simulink model "Rozmyty_fuzzy_controler"  (R2017b)
settings: Solver=ode1  StartTime=0.0  StopTime=4  FixedStep=0.001  RelTol=1e-3
values from neighbouring files (symbols this model uses):
  Te = 0.001    [Dane_rozmyte.m]
  Tm = 0.2    [Dane_rozmyte.m]
libraries: fuzblock x6
settings Model: Creator=kamil  LastModifiedBy=kamil

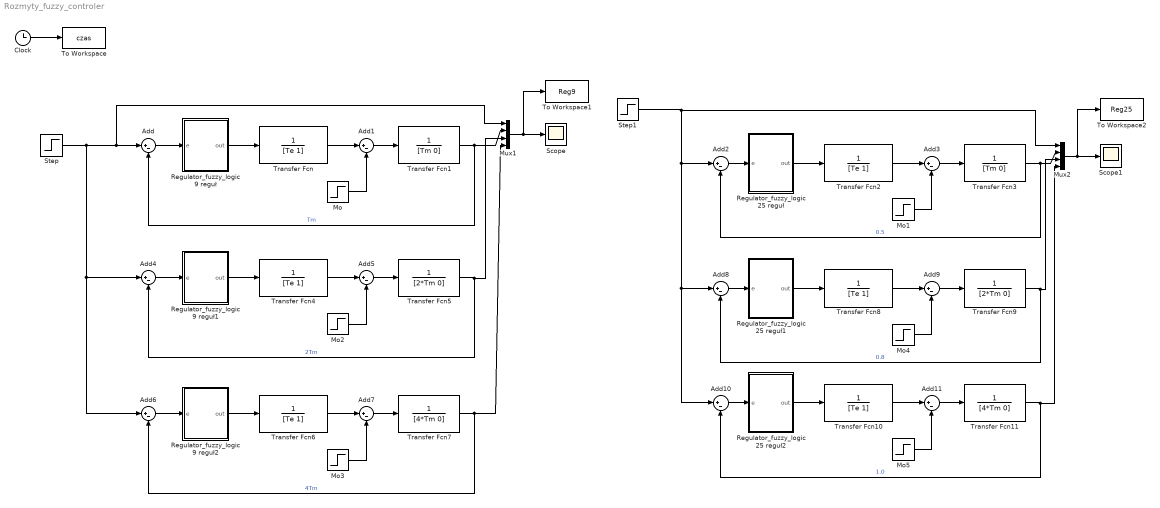
== system Rozmyty_fuzzy_controler ==
  Add{,1..11} (12 alike) : Sum  Inputs=|+-
  Clock : Clock
  Mo{,1..5} (6 alike) : Step  Time=2  After=0.5  SampleTime=0
  Mux1 : Mux
  Mux2 : Mux
  Regulator_fuzzy_logic 25 reguł : Subsystem
  Regulator_fuzzy_logic 25 reguł1 : Subsystem
  Regulator_fuzzy_logic 25 reguł2 : Subsystem
  Regulator_fuzzy_logic 9 reguł : Subsystem
  Regulator_fuzzy_logic 9 reguł1 : Subsystem
  Regulator_fuzzy_logic 9 reguł2 : Subsystem
  Scope : Scope
  Scope1 : Scope
  Step : Step  After=0.25  SampleTime=0
  Step1 : Step  After=0.25  SampleTime=0
  To Workspace : ToWorkspace  VariableName=czas  SampleTime=-1
  To Workspace1 : ToWorkspace  VariableName=Reg9  SampleTime=-1
  To Workspace2 : ToWorkspace  VariableName=Reg25  SampleTime=-1
  Transfer Fcn{,2,4,6,8,10} (6 alike) : TransferFcn  Denominator=[Te 1]
  Transfer Fcn1 : TransferFcn  Denominator=[Tm 0]
  Transfer Fcn11 : TransferFcn  Denominator=[4*Tm 0]
  Transfer Fcn3 : TransferFcn  Denominator=[Tm 0]
  Transfer Fcn5 : TransferFcn  Denominator=[2*Tm 0]
  Transfer Fcn7 : TransferFcn  Denominator=[4*Tm 0]
  Transfer Fcn9 : TransferFcn  Denominator=[2*Tm 0]
  wires:
  Add1/1 -> Transfer Fcn1/1
  Mo/1 -> Add1/2
  Transfer Fcn/1 -> Add1/1
  Transfer Fcn1/1 -> Mux1/2, Add/2  "Tm"
  Mux1/1 -> To Workspace1/1, Scope/1
  Add/1 -> Regulator_fuzzy_logic 9 reguł/1(e)
  Regulator_fuzzy_logic 9 reguł/1(out) -> Transfer Fcn/1
  Clock/1 -> To Workspace/1
  Mo1/1 -> Add3/2
  Add2/1 -> Regulator_fuzzy_logic 25 reguł/1(e)
  Transfer Fcn3/1 -> Mux2/2, Add2/2  "0.5"
  Mux2/1 -> To Workspace2/1, Scope1/1
  Add3/1 -> Transfer Fcn3/1
  Regulator_fuzzy_logic 25 reguł/1(out) -> Transfer Fcn2/1
  Transfer Fcn2/1 -> Add3/1
  Mo2/1 -> Add5/2
  Add4/1 -> Regulator_fuzzy_logic 9 reguł1/1(e)
  Add5/1 -> Transfer Fcn5/1
  Regulator_fuzzy_logic 9 reguł1/1(out) -> Transfer Fcn4/1
  Transfer Fcn4/1 -> Add5/1
  Transfer Fcn5/1 -> Mux1/3, Add4/2  "2Tm"
  Mo3/1 -> Add7/2
  Add6/1 -> Regulator_fuzzy_logic 9 reguł2/1(e)
  Add7/1 -> Transfer Fcn7/1
  Regulator_fuzzy_logic 9 reguł2/1(out) -> Transfer Fcn6/1
  Transfer Fcn6/1 -> Add7/1
  Transfer Fcn7/1 -> Mux1/4, Add6/2  "4Tm"
  Step/1 -> Add6/1, Add4/1, Mux1/1, Add/1
  Transfer Fcn9/1 -> Mux2/3, Add8/2  "0.8"
  Transfer Fcn8/1 -> Add9/1
  Regulator_fuzzy_logic 25 reguł1/1(out) -> Transfer Fcn8/1
  Add9/1 -> Transfer Fcn9/1
  Mo4/1 -> Add9/2
  Add8/1 -> Regulator_fuzzy_logic 25 reguł1/1(e)
  Transfer Fcn11/1 -> Mux2/4, Add10/2  "1.0"
  Transfer Fcn10/1 -> Add11/1
  Regulator_fuzzy_logic 25 reguł2/1(out) -> Transfer Fcn10/1
  Add11/1 -> Transfer Fcn11/1
  Mo5/1 -> Add11/2
  Step1/1 -> Mux2/1, Add10/1, Add8/1, Add2/1
  Add10/1 -> Regulator_fuzzy_logic 25 reguł2/1(e)

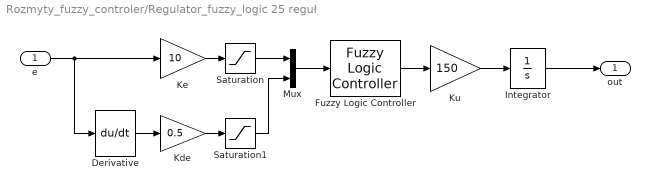
== system Rozmyty_fuzzy_controler/Regulator_fuzzy_logic 25 reguł ==
  e : Inport
  Derivative : Derivative
  Fuzzy Logic Controller : fuzblock/Fuzzy Logic  Controller  FIS=Reg_5  OutputSampleNumber=101  DataType=double  FuzzifiedInputs=off  RuleFiringStrengths=off  RuleOutputs=off  AggregatedOutputs=off  SimulateUsing=Interpreted execution
  Integrator : Integrator
  Kde : Gain  Gain=0.5
  Ke : Gain  Gain=10
  Ku : Gain  Gain=150
  Mux : Mux  Inputs=2
  Saturation : Saturate  UpperLimit=1  LowerLimit=-1
  Saturation1 : Saturate  UpperLimit=1  LowerLimit=-1
  out : Outport
  wires:
  Integrator/1 -> out/1
  Mux/1 -> Fuzzy Logic Controller/1
  Ke/1 -> Saturation/1
  Kde/1 -> Saturation1/1
  Derivative/1 -> Kde/1
  Saturation/1 -> Mux/1
  Saturation1/1 -> Mux/2
  e/1 -> Derivative/1, Ke/1
  Ku/1 -> Integrator/1
  Fuzzy Logic Controller/1 -> Ku/1

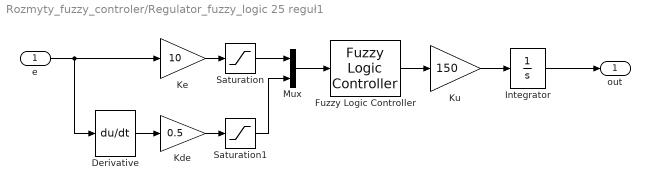
== system Rozmyty_fuzzy_controler/Regulator_fuzzy_logic 25 reguł1 ==
  e : Inport
  Derivative : Derivative
  Fuzzy Logic Controller : fuzblock/Fuzzy Logic  Controller  FIS=Reg_5  OutputSampleNumber=101  DataType=double  FuzzifiedInputs=off  RuleFiringStrengths=off  RuleOutputs=off  AggregatedOutputs=off  SimulateUsing=Interpreted execution
  Integrator : Integrator
  Kde : Gain  Gain=0.5
  Ke : Gain  Gain=10
  Ku : Gain  Gain=150
  Mux : Mux  Inputs=2
  Saturation : Saturate  UpperLimit=1  LowerLimit=-1
  Saturation1 : Saturate  UpperLimit=1  LowerLimit=-1
  out : Outport
  wires:
  Integrator/1 -> out/1
  Mux/1 -> Fuzzy Logic Controller/1
  Ke/1 -> Saturation/1
  Kde/1 -> Saturation1/1
  Derivative/1 -> Kde/1
  Saturation/1 -> Mux/1
  Saturation1/1 -> Mux/2
  e/1 -> Derivative/1, Ke/1
  Ku/1 -> Integrator/1
  Fuzzy Logic Controller/1 -> Ku/1

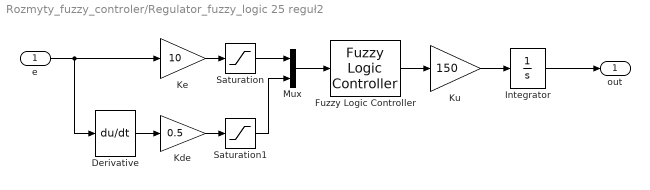
== system Rozmyty_fuzzy_controler/Regulator_fuzzy_logic 25 reguł2 ==
  e : Inport
  Derivative : Derivative
  Fuzzy Logic Controller : fuzblock/Fuzzy Logic  Controller  FIS=Reg_5  OutputSampleNumber=101  DataType=double  FuzzifiedInputs=off  RuleFiringStrengths=off  RuleOutputs=off  AggregatedOutputs=off  SimulateUsing=Interpreted execution
  Integrator : Integrator
  Kde : Gain  Gain=0.5
  Ke : Gain  Gain=10
  Ku : Gain  Gain=150
  Mux : Mux  Inputs=2
  Saturation : Saturate  UpperLimit=1  LowerLimit=-1
  Saturation1 : Saturate  UpperLimit=1  LowerLimit=-1
  out : Outport
  wires:
  Integrator/1 -> out/1
  Mux/1 -> Fuzzy Logic Controller/1
  Ke/1 -> Saturation/1
  Kde/1 -> Saturation1/1
  Derivative/1 -> Kde/1
  Saturation/1 -> Mux/1
  Saturation1/1 -> Mux/2
  e/1 -> Derivative/1, Ke/1
  Ku/1 -> Integrator/1
  Fuzzy Logic Controller/1 -> Ku/1

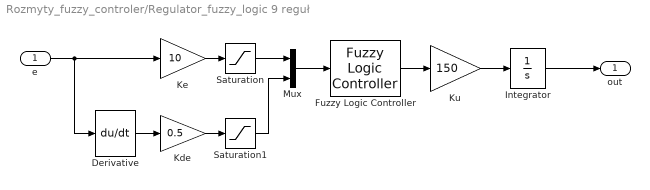
== system Rozmyty_fuzzy_controler/Regulator_fuzzy_logic 9 reguł ==
  e : Inport
  Derivative : Derivative
  Fuzzy Logic Controller : fuzblock/Fuzzy Logic  Controller  FIS=Reg_3  OutputSampleNumber=101  DataType=double  FuzzifiedInputs=off  RuleFiringStrengths=off  RuleOutputs=off  AggregatedOutputs=off  SimulateUsing=Interpreted execution
  Integrator : Integrator
  Kde : Gain  Gain=0.5
  Ke : Gain  Gain=10
  Ku : Gain  Gain=150
  Mux : Mux  Inputs=2
  Saturation : Saturate  UpperLimit=1  LowerLimit=-1
  Saturation1 : Saturate  UpperLimit=1  LowerLimit=-1
  out : Outport
  wires:
  Integrator/1 -> out/1
  Mux/1 -> Fuzzy Logic Controller/1
  Ke/1 -> Saturation/1
  Kde/1 -> Saturation1/1
  Derivative/1 -> Kde/1
  Saturation/1 -> Mux/1
  Saturation1/1 -> Mux/2
  e/1 -> Derivative/1, Ke/1
  Ku/1 -> Integrator/1
  Fuzzy Logic Controller/1 -> Ku/1

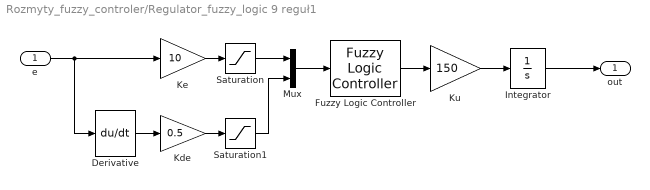
== system Rozmyty_fuzzy_controler/Regulator_fuzzy_logic 9 reguł1 ==
  e : Inport
  Derivative : Derivative
  Fuzzy Logic Controller : fuzblock/Fuzzy Logic  Controller  FIS=Reg_3  OutputSampleNumber=101  DataType=double  FuzzifiedInputs=off  RuleFiringStrengths=off  RuleOutputs=off  AggregatedOutputs=off  SimulateUsing=Interpreted execution
  Integrator : Integrator
  Kde : Gain  Gain=0.5
  Ke : Gain  Gain=10
  Ku : Gain  Gain=150
  Mux : Mux  Inputs=2
  Saturation : Saturate  UpperLimit=1  LowerLimit=-1
  Saturation1 : Saturate  UpperLimit=1  LowerLimit=-1
  out : Outport
  wires:
  Integrator/1 -> out/1
  Mux/1 -> Fuzzy Logic Controller/1
  Ke/1 -> Saturation/1
  Kde/1 -> Saturation1/1
  Derivative/1 -> Kde/1
  Saturation/1 -> Mux/1
  Saturation1/1 -> Mux/2
  e/1 -> Derivative/1, Ke/1
  Ku/1 -> Integrator/1
  Fuzzy Logic Controller/1 -> Ku/1

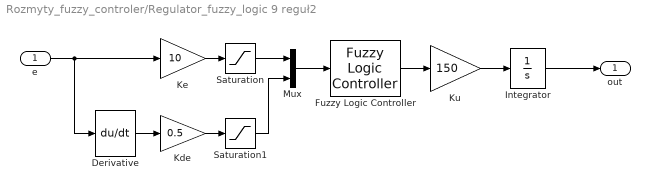
== system Rozmyty_fuzzy_controler/Regulator_fuzzy_logic 9 reguł2 ==
  e : Inport
  Derivative : Derivative
  Fuzzy Logic Controller : fuzblock/Fuzzy Logic  Controller  FIS=Reg_3  OutputSampleNumber=101  DataType=double  FuzzifiedInputs=off  RuleFiringStrengths=off  RuleOutputs=off  AggregatedOutputs=off  SimulateUsing=Interpreted execution
  Integrator : Integrator
  Kde : Gain  Gain=0.5
  Ke : Gain  Gain=10
  Ku : Gain  Gain=150
  Mux : Mux  Inputs=2
  Saturation : Saturate  UpperLimit=1  LowerLimit=-1
  Saturation1 : Saturate  UpperLimit=1  LowerLimit=-1
  out : Outport
  wires:
  Integrator/1 -> out/1
  Mux/1 -> Fuzzy Logic Controller/1
  Ke/1 -> Saturation/1
  Kde/1 -> Saturation1/1
  Derivative/1 -> Kde/1
  Saturation/1 -> Mux/1
  Saturation1/1 -> Mux/2
  e/1 -> Derivative/1, Ke/1
  Ku/1 -> Integrator/1
  Fuzzy Logic Controller/1 -> Ku/1
